simulink model "Pioneer_Aircraft_Model"  (Simulink 4.1.1)
settings: Solver=ode4  SolverMode=SingleTasking  StartTime=0.0  StopTime=1600  FixedStep=Flight_TimeStep  MaxStep=0.1  MinStep=0.001  RelTol=1e-3
undefined symbols (not defined in the file): Flight_TargetPoints
libraries: simulink3 x1, AeroLib x1
settings Model: LastModifiedBy=pascaleg  InitialStep=0.01  ExternalInput=[0, utin']  SaveTime=off  SaveOutput=off  InitialState=xtin  MaxDataPoints=5000  Decimation=10  OptimizeBlockIOStorage=off  BufferReuse=off  BlockReductionOpt=off

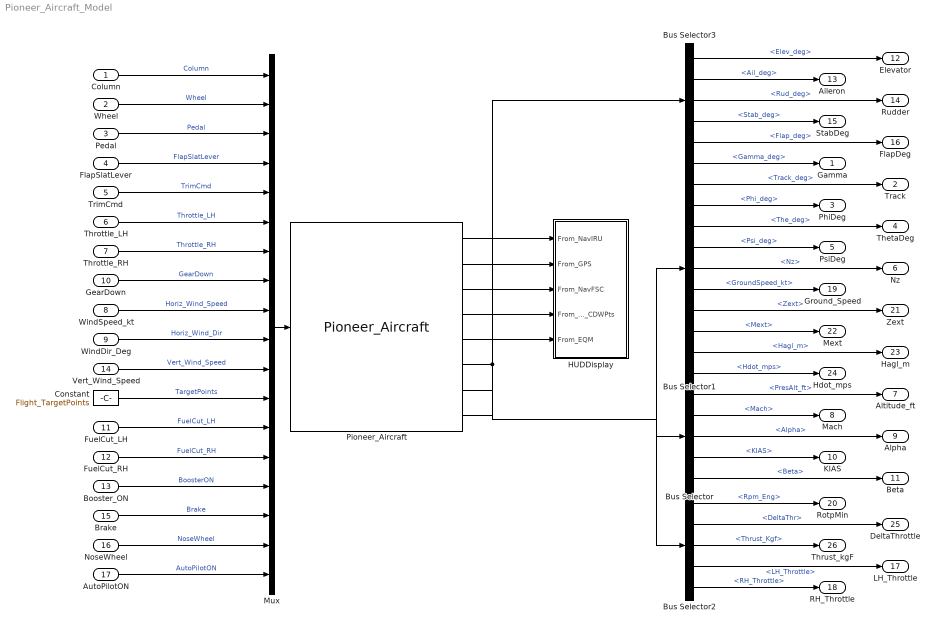
== system Pioneer_Aircraft_Model ==
  Column : Inport  Port=1  LatchInput=off
  Wheel : Inport  Port=2  LatchInput=off
  Pedal : Inport  Port=3  LatchInput=off
  FlapSlatLever : Inport  Port=4  LatchInput=off
  TrimCmd : Inport  Port=5  LatchInput=off
  Throttle_LH : Inport  Port=6  LatchInput=off
  Throttle_RH : Inport  Port=7  LatchInput=off
  WindSpeed_kt : Inport  Port=8  LatchInput=off
  WindDir_Deg : Inport  Port=9  LatchInput=off
  GearDown : Inport  Port=10  LatchInput=off
  FuelCut_LH : Inport  Port=11  LatchInput=off
  FuelCut_RH : Inport  Port=12  LatchInput=off
  Booster_ON : Inport  Port=13  LatchInput=off
  Vert_Wind_Speed : Inport  Port=14  LatchInput=off
  Brake : Inport  Port=15  LatchInput=off
  NoseWheel : Inport  Port=16  LatchInput=off
  AutoPilotON : Inport  Port=17  LatchInput=off
  Bus Selector : BusSelector  OutputSignals=PresAlt_ft,Mach,Alpha,KIAS,Beta  MuxedOutput=off
  Bus Selector1 : BusSelector  OutputSignals=Gamma_deg,Track_deg,Phi_deg,The_deg,Psi_deg,Nz,GroundSpeed_kt,Zext,Mext,Hagl_m,Hdot_mps  MuxedOutput=off
  Bus Selector2 : BusSelector  OutputSignals=Rpm_Eng,DeltaThr,Thrust_Kgf,LH_Throttle,RH_Throttle  MuxedOutput=off
  Bus Selector3 : BusSelector  OutputSignals=Elev_deg,Ail_deg,Rud_deg,Stab_deg,Flap_deg  MuxedOutput=off
  Constant : Constant  Value=Flight_TargetPoints
  HUDDisplay : Subsystem
      settings: RTWFcnNameOpts=Auto  RTWFileNameOpts=Auto
  Mux : Mux  Inputs=18
  Pioneer_Aircraft : AeroLib/Aircraft/Pioneer_Aircraft
  Gamma : Outport  Port=1
  Track : Outport  Port=2
  PhiDeg : Outport  Port=3
  ThetaDeg : Outport  Port=4
  PsiDeg : Outport  Port=5
  Nz : Outport  Port=6
  Altitude_ft : Outport  Port=7
  Mach : Outport  Port=8
  Alpha : Outport  Port=9
  KIAS : Outport  Port=10
  Beta : Outport  Port=11
  Elevator : Outport  Port=12
  Aileron : Outport  Port=13
  Rudder : Outport  Port=14
  StabDeg : Outport  Port=15
  FlapDeg : Outport  Port=16
  LH_Throttle : Outport  Port=17
  RH_Throttle : Outport  Port=18
  Ground_Speed : Outport  Port=19
  RotpMin : Outport  Port=20
  Zext : Outport  Port=21
  Mext : Outport  Port=22
  Hagl_m : Outport  Port=23
  Hdot_mps : Outport  Port=24
  DeltaThrottle : Outport  Port=25
  Thrust_kgF : Outport  Port=26
  wires:
  Column/1 -> Mux/1  "Column"
  Wheel/1 -> Mux/2  "Wheel"
  Pedal/1 -> Mux/3  "Pedal"
  FlapSlatLever/1 -> Mux/4  "FlapSlatLever"
  Throttle_LH/1 -> Mux/6  "Throttle_LH"
  TrimCmd/1 -> Mux/5  "TrimCmd"
  Throttle_RH/1 -> Mux/7  "Throttle_RH"
  WindSpeed_kt/1 -> Mux/9  "Horiz_Wind_Speed"
  WindDir_Deg/1 -> Mux/10  "Horiz_Wind_Dir"
  Mux/1 -> Pioneer_Aircraft/1
  Bus Selector/2 -> Mach/1  "<Mach>"
  Bus Selector/3 -> Alpha/1  "<Alpha>"
  Bus Selector/4 -> KIAS/1  "<KIAS>"
  Bus Selector/1 -> Altitude_ft/1  "<PresAlt_ft>"
  Bus Selector1/5 -> PsiDeg/1  "<Psi_deg>"
  Bus Selector1/4 -> ThetaDeg/1  "<The_deg>"
  Bus Selector1/1 -> Gamma/1  "<Gamma_deg>"
  Bus Selector1/3 -> PhiDeg/1  "<Phi_deg>"
  Bus Selector1/2 -> Track/1  "<Track_deg>"
  Bus Selector/5 -> Beta/1  "<Beta>"
  Bus Selector3/1 -> Elevator/1  "<Elev_deg>"
  Bus Selector3/2 -> Aileron/1  "<Ail_deg>"
  Bus Selector3/3 -> Rudder/1  "<Rud_deg>"
  Bus Selector3/4 -> StabDeg/1  "<Stab_deg>"
  Bus Selector1/6 -> Nz/1  "<Nz>"
  Bus Selector3/5 -> FlapDeg/1  "<Flap_deg>"
  Bus Selector1/7 -> Ground_Speed/1  "<GroundSpeed_kt>"
  GearDown/1 -> Mux/8  "GearDown"
  Bus Selector2/1 -> RotpMin/1  "<Rpm_Eng>"
  Booster_ON/1 -> Mux/15  "BoosterON"
  FuelCut_RH/1 -> Mux/14  "FuelCut_RH"
  FuelCut_LH/1 -> Mux/13  "FuelCut_LH"
  Constant/1 -> Mux/12  "TargetPoints"
  Vert_Wind_Speed/1 -> Mux/11  "Vert_Wind_Speed"
  Brake/1 -> Mux/16  "Brake"
  NoseWheel/1 -> Mux/17  "NoseWheel"
  Bus Selector1/8 -> Zext/1  "<Zext>"
  Bus Selector1/9 -> Mext/1  "<Mext>"
  Bus Selector1/10 -> Hagl_m/1  "<Hagl_m>"
  Bus Selector1/11 -> Hdot_mps/1  "<Hdot_mps>"
  AutoPilotON/1 -> Mux/18  "AutoPilotON"
  Bus Selector2/2 -> DeltaThrottle/1  "<DeltaThr>"
  Pioneer_Aircraft/5 -> Bus Selector3/1
  Pioneer_Aircraft/6 -> Bus Selector1/1, HUDDisplay/5(From_EQM)
  Pioneer_Aircraft/7 -> Bus Selector/1
  Pioneer_Aircraft/8 -> Bus Selector2/1
  Bus Selector2/3 -> Thrust_kgF/1  "<Thrust_Kgf>"
  Pioneer_Aircraft/1 -> HUDDisplay/1(From_NavIRU)
  Pioneer_Aircraft/2 -> HUDDisplay/2(From_GPS)
  Pioneer_Aircraft/3 -> HUDDisplay/3(From_NavFSC)
  Pioneer_Aircraft/4 -> HUDDisplay/4(From_AP_CDWPts)
  Bus Selector2/5 -> RH_Throttle/1  "<RH_Throttle>"
  Bus Selector2/4 -> LH_Throttle/1  "<LH_Throttle>"

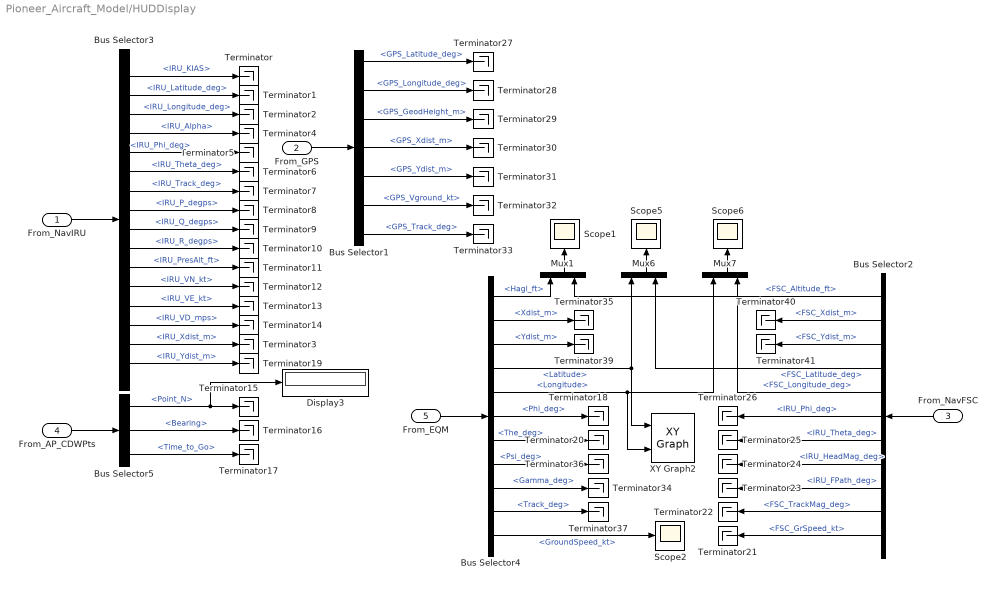
== system Pioneer_Aircraft_Model/HUDDisplay ==
  From_NavIRU : Inport  Port=1  LatchInput=off
  From_GPS : Inport  Port=2  LatchInput=off
  From_NavFSC : Inport  Orientation=left  Port=3  LatchInput=off
  From_AP_CDWPts : Inport  Port=4  LatchInput=off
  From_EQM : Inport  Port=5  LatchInput=off
  Bus Selector1 : BusSelector  OutputSignals=GPS_Latitude_deg,GPS_Longitude_deg,GPS_GeodHeight_m,GPS_Xdist_m,GPS_Ydist_m,GPS_Vground_kt,GPS_Track_deg  MuxedOutput=off
  Bus Selector2 : BusSelector  Orientation=left  OutputSignals=FSC_Altitude_ft,FSC_Xdist_m,FSC_Ydist_m,FSC_Latitude_deg,FSC_Longitude_deg,IRU_Phi_deg,IRU_Theta_deg,IRU_HeadMag_deg,IRU_FPath_deg,FSC_TrackMag_deg,FSC_GrSpeed_kt  MuxedOutput=off
  Bus Selector3 : BusSelector  OutputSignals=IRU_KIAS,IRU_Latitude_deg,IRU_Longitude_deg,IRU_Alpha,IRU_Phi_deg,IRU_Theta_deg,IRU_Track_deg,IRU_P_degps,IRU_Q_degps,IRU_R_degps,IRU_PresAlt_ft,IRU_VN_kt,IRU_VE_kt,IRU_VD_mps,IRU_Xdist_m,IRU_Ydist_m  MuxedOutput=off
  Bus Selector4 : BusSelector  OutputSignals=Hagl_ft,Xdist_m,Ydist_m,Latitude,Longitude,Phi_deg,The_deg,Psi_deg,Gamma_deg,Track_deg,GroundSpeed_kt  MuxedOutput=off
  Bus Selector5 : BusSelector  OutputSignals=Point_N,Bearing,Time_to_Go  MuxedOutput=off
  Display3 : Display
      settings: Format=short  Decimation=50
  Mux1 : Mux  Orientation=up  Inputs=2
  Mux6 : Mux  Orientation=up  Inputs=2
  Mux7 : Mux  Orientation=up  Inputs=2
  Scope{1..2,5..6} (4 alike) : Scope
      Scope1 settings: Orientation=up  TimeRange=auto  YMin=495  YMax=565  SaveToWorkspace=off  SaveName=ScopeData3  LimitDataPoints=on  MaxDataPoints=5000  Decimation=10
      Scope2 settings: TimeRange=auto  YMin=65  YMax=120  SaveToWorkspace=off  LimitDataPoints=on  MaxDataPoints=5000  Decimation=10
      Scope5 settings: Orientation=up  TimeRange=auto  YMin=29.785  YMax=29.8075  SaveToWorkspace=off  SaveName=ScopeData6  LimitDataPoints=on  MaxDataPoints=5000  Decimation=10
      Scope6 settings: Orientation=up  TimeRange=auto  YMin=150.695  YMax=150.705  SaveToWorkspace=off  SaveName=ScopeData7  LimitDataPoints=on  MaxDataPoints=5000  Decimation=10
  Terminator{,1..37,39..41} (41 alike) : Terminator
  XY Graph2 : simulink3/Sinks/XY Graph  xmin=30  xmax=31  ymin=150  ymax=151  st=-1
  wires:
  Bus Selector3/16 -> Terminator19/1  "<IRU_Ydist_m>"
  Bus Selector3/15 -> Terminator3/1  "<IRU_Xdist_m>"
  Bus Selector5/3 -> Terminator17/1  "<Time_to_Go>"
  Bus Selector5/2 -> Terminator16/1  "<Bearing>"
  Bus Selector5/1 -> Terminator15/1, Display3/1  "<Point_N>"
  Bus Selector3/14 -> Terminator14/1  "<IRU_VD_mps>"
  Bus Selector3/13 -> Terminator13/1  "<IRU_VE_kt>"
  Bus Selector3/12 -> Terminator12/1  "<IRU_VN_kt>"
  Bus Selector3/11 -> Terminator11/1  "<IRU_PresAlt_ft>"
  Bus Selector3/10 -> Terminator10/1  "<IRU_R_degps>"
  Bus Selector3/9 -> Terminator9/1  "<IRU_Q_degps>"
  Bus Selector3/8 -> Terminator8/1  "<IRU_P_degps>"
  Bus Selector3/7 -> Terminator7/1  "<IRU_Track_deg>"
  Bus Selector3/6 -> Terminator6/1  "<IRU_Theta_deg>"
  Bus Selector3/5 -> Terminator5/1  "<IRU_Phi_deg>"
  Bus Selector3/4 -> Terminator4/1  "<IRU_Alpha>"
  Bus Selector3/3 -> Terminator2/1  "<IRU_Longitude_deg>"
  Bus Selector3/1 -> Terminator/1  "<IRU_KIAS>"
  From_NavIRU/1 -> Bus Selector3/1
  From_AP_CDWPts/1 -> Bus Selector5/1
  From_NavFSC/1 -> Bus Selector2/1
  From_GPS/1 -> Bus Selector1/1
  Bus Selector1/1 -> Terminator27/1  "<GPS_Latitude_deg>"
  Bus Selector1/2 -> Terminator28/1  "<GPS_Longitude_deg>"
  Bus Selector1/3 -> Terminator29/1  "<GPS_GeodHeight_m>"
  Bus Selector1/4 -> Terminator30/1  "<GPS_Xdist_m>"
  Bus Selector1/5 -> Terminator31/1  "<GPS_Ydist_m>"
  Bus Selector1/6 -> Terminator32/1  "<GPS_Vground_kt>"
  Bus Selector1/7 -> Terminator33/1  "<GPS_Track_deg>"
  Bus Selector3/2 -> Terminator1/1  "<IRU_Latitude_deg>"
  From_EQM/1 -> Bus Selector4/1
  Mux1/1 -> Scope1/1
  Bus Selector4/1 -> Mux1/1  "<Hagl_ft>"
  Bus Selector4/4 -> Mux6/1, XY Graph2/1  "<Latitude>"
  Bus Selector4/5 -> Mux7/1, XY Graph2/2  "<Longitude>"
  Bus Selector4/6 -> Terminator18/1  "<Phi_deg>"
  Bus Selector4/7 -> Terminator20/1  "<The_deg>"
  Bus Selector4/8 -> Terminator36/1  "<Psi_deg>"
  Bus Selector4/9 -> Terminator34/1  "<Gamma_deg>"
  Bus Selector4/10 -> Terminator37/1  "<Track_deg>"
  Bus Selector4/11 -> Scope2/1  "<GroundSpeed_kt>"
  Bus Selector2/1 -> Mux1/2  "<FSC_Altitude_ft>"
  Mux6/1 -> Scope5/1
  Mux7/1 -> Scope6/1
  Bus Selector2/4 -> Mux6/2  "<FSC_Latitude_deg>"
  Bus Selector2/5 -> Mux7/2  "<FSC_Longitude_deg>"
  Bus Selector2/11 -> Terminator21/1  "<FSC_GrSpeed_kt>"
  Bus Selector2/10 -> Terminator22/1  "<FSC_TrackMag_deg>"
  Bus Selector2/9 -> Terminator23/1  "<IRU_FPath_deg>"
  Bus Selector2/8 -> Terminator24/1  "<IRU_HeadMag_deg>"
  Bus Selector2/7 -> Terminator25/1  "<IRU_Theta_deg>"
  Bus Selector2/6 -> Terminator26/1  "<IRU_Phi_deg>"
  Bus Selector4/2 -> Terminator35/1  "<Xdist_m>"
  Bus Selector4/3 -> Terminator39/1  "<Ydist_m>"
  Bus Selector2/2 -> Terminator40/1  "<FSC_Xdist_m>"
  Bus Selector2/3 -> Terminator41/1  "<FSC_Ydist_m>"
